simulink model "hf1simuAQCOKQ"  (R2023a)
settings: Solver=VariableStepAuto  StartTime=0.0  StopTime=20  RelTol=1e-3
values from neighbouring files (symbols this model uses):
  den = [m1*m2 (m1+m2)*b (m1+m2)*k]    [hf1AQCOKQ.m]
  num = m1    (= 1)    [hf1AQCOKQ.m]
  sigma = 0.01    [hf1AQCOKQ.m]
  U = 6    [hf1AQCOKQ.m]
  w = 1.2    [hf1AQCOKQ.m]
settings Model: Creator=simon  LastModifiedBy=simon

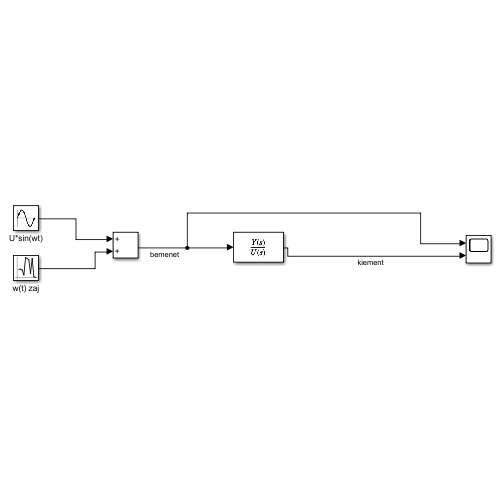
[thumbnail: Simulink's stored preview of the top-level diagram]
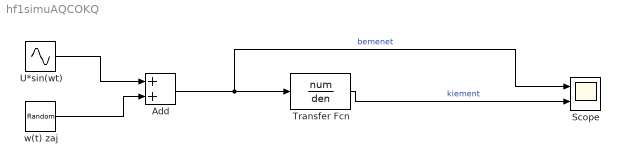
== system hf1simuAQCOKQ ==
  Add : Sum
  Scope : Scope  NumInputPorts=2
  Transfer Fcn : TransferFcn  Numerator=num  Denominator=den
  U*sin(wt) : Sin  Amplitude=U  Frequency=w  SampleTime=0
  w(t) zaj : RandomNumber  Variance=sigma  SampleTime=0.1
  wires:
  U*sin(wt)/1 -> Add/1
  w(t) zaj/1 -> Add/2
  Add/1 -> Scope/1, Transfer Fcn/1  "bemenet"
  Transfer Fcn/1 -> Scope/2  "kiement"
